simulink model "z2"  (R2023a)
settings: Solver=VariableStepAuto  StartTime=0.0  StopTime=10.0  RelTol=1e-3
libraries: fl_lib x10, nesl_utility x7, simulink_extras x2, ee_lib x2
settings Model: Creator=Artyom  LastModifiedBy=Пажылой ай3

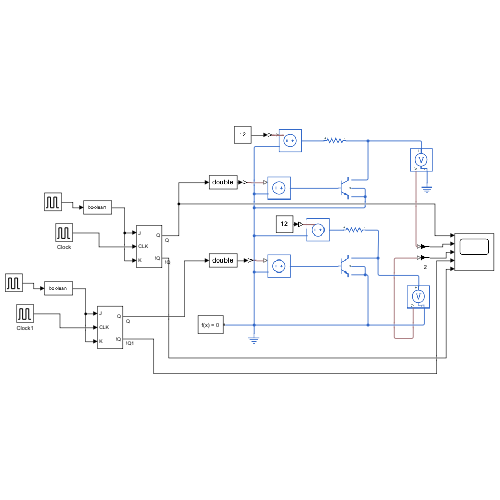
[thumbnail: Simulink's stored preview of the top-level diagram]
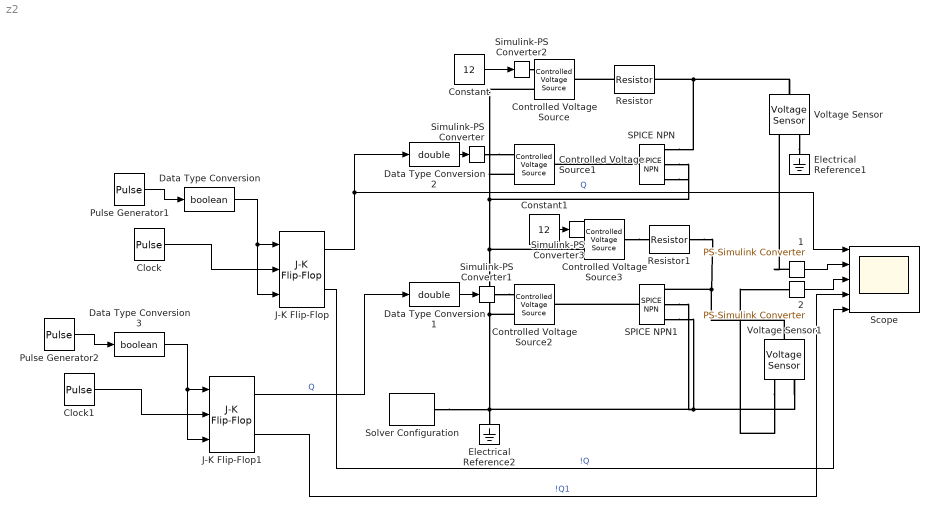
== system z2 ==
  1 : nesl_utility/PS-Simulink Converter  PhysicalDomain=network_engine_domain  SubClassName=ps_output  LeftPortType=input  RightPortType=output  PseudoPeriodic=off  Frequencies=[]  VectorFormat=inherit  Unit=inherit  AffineConversion=off
  2 : nesl_utility/PS-Simulink Converter  PhysicalDomain=network_engine_domain  SubClassName=ps_output  LeftPortType=input  RightPortType=output  PseudoPeriodic=off  Frequencies=[]  VectorFormat=inherit  Unit=inherit  AffineConversion=off
  Clock : DiscretePulseGenerator  PulseType=Time based  Period=1  PulseWidth=50
  Clock1 : DiscretePulseGenerator  PulseType=Time based  Period=1  PulseWidth=50  PhaseDelay=1
  Constant : Constant  Value=12
  Constant1 : Constant  Value=12
  Controlled Voltage Source{,1..3} (4 alike) : fl_lib/Electrical/Electrical Sources/Controlled Voltage Source
  Data Type Conversion : DataTypeConversion  OutDataTypeStr=boolean  SaturateOnIntegerOverflow=off  RndMeth=Floor
  Data Type Conversion1 : DataTypeConversion  OutDataTypeStr=double  SaturateOnIntegerOverflow=off  RndMeth=Floor
  Data Type Conversion2 : DataTypeConversion  OutDataTypeStr=double  SaturateOnIntegerOverflow=off  RndMeth=Floor
  Data Type Conversion3 : DataTypeConversion  OutDataTypeStr=boolean  SaturateOnIntegerOverflow=off  RndMeth=Floor
  Electrical Reference1 : fl_lib/Electrical/Electrical Elements/Electrical Reference
  Electrical Reference2 : fl_lib/Electrical/Electrical Elements/Electrical Reference
  J-K Flip-Flop : simulink_extras/Flip Flops/J-K Flip-Flop  initial_condition=0
  J-K Flip-Flop1 : simulink_extras/Flip Flops/J-K Flip-Flop  initial_condition=0
  Pulse Generator1 : DiscretePulseGenerator  PulseType=Time based  Period=0.035  PulseWidth=50
  Pulse Generator2 : DiscretePulseGenerator  PulseType=Time based  Period=0.035  PulseWidth=50
  Resistor : fl_lib/Electrical/Electrical Elements/Resistor  R=60 Ohm  i_specify=off  i_priority=None  i=0 A  i_nominal_specify=off  i_nominal_unit=A  i_nominal_value=1  v_specify=off  v_priority=None  v=0 V  v_nominal_specify=off  v_nominal_unit=V  v_nominal_value=1
  Resistor1 : fl_lib/Electrical/Electrical Elements/Resistor  R=60 Ohm  i_specify=off  i_priority=None  i=0 A  i_nominal_specify=off  i_nominal_unit=A  i_nominal_value=1  v_specify=off  v_priority=None  v=0 V  v_nominal_specify=off  v_nominal_unit=V  v_nominal_value=1
  SPICE NPN : ee_lib/Additional Components/SPICE Semiconductors/SPICE NPN  AREA=1.0 m^2  SCALE=1  IS=1.0e-16 A/m^2  BF=100.0  NF=1  VAF=Inf V  IKF=Inf A/m^2  ISE=0 A/m^2  NE=1.5  BR=1  NR=1  VAR=Inf V  IKR=Inf A/m^2  ISC=0 A/m^2  NC=2  RB=1 Ohm*m^2  IRB=Inf A/m^2  RBM=0 Ohm*m^2  RE=1e-4 Ohm*m^2  RC=0.01 Ohm*m^2  C_param=1  FC=0.5  IC_given=1  ICVBE=0 V  ICVCE=0 V  CJE=0 F/m^2  VJE=0.75 V  MJE=0.33  TF=0 s  XTF=0  VTF=Inf V  ITF=0 A/m^2  CJC=0 F/m^2  VJC=0.75 V  MJC=0.33  XCJC=1  TR=0 s  CJS=0 F/m^2  VJS=0.75 V  MJS=0  T_param=1  XTB=0  EG=1.11 eV  XTI=3  TFIXED=300.15 K  TMEAS=300.15 K  TOFFSET=0 K
      settings: InternalSimscapePortConfiguration="{\"Bottom\":[],\"Left\":[{\"id\":\"bx\",\"label\":\"\",\"type\":\"foundation.electrical.electrical\"}],\"Right\":[{\"id\":\"cx\",\"label\":\"\",\"type\":\"foundation.electrical.electrical\"},{\"id\":\"sx\",\"label\":\"s\",\"type\":\"foundation.electrical.electrical\"},{\"id\":\"ex\",\"label\":\"\",\"type\":\"foundation.electrical.electrical\"}],\"Top\":[]}"
  SPICE NPN1 : ee_lib/Additional Components/SPICE Semiconductors/SPICE NPN  AREA=1.0 m^2  SCALE=1  IS=1.0e-16 A/m^2  BF=100.0  NF=1  VAF=Inf V  IKF=Inf A/m^2  ISE=0 A/m^2  NE=1.5  BR=1  NR=1  VAR=Inf V  IKR=Inf A/m^2  ISC=0 A/m^2  NC=2  RB=1 Ohm*m^2  IRB=Inf A/m^2  RBM=0 Ohm*m^2  RE=1e-4 Ohm*m^2  RC=0.01 Ohm*m^2  C_param=1  FC=0.5  IC_given=1  ICVBE=0 V  ICVCE=0 V  CJE=0 F/m^2  VJE=0.75 V  MJE=0.33  TF=0 s  XTF=0  VTF=Inf V  ITF=0 A/m^2  CJC=0 F/m^2  VJC=0.75 V  MJC=0.33  XCJC=1  TR=0 s  CJS=0 F/m^2  VJS=0.75 V  MJS=0  T_param=1  XTB=0  EG=1.11 eV  XTI=3  TFIXED=300.15 K  TMEAS=300.15 K  TOFFSET=0 K
      settings: InternalSimscapePortConfiguration="{\"Bottom\":[],\"Left\":[{\"id\":\"bx\",\"label\":\"\",\"type\":\"foundation.electrical.electrical\"}],\"Right\":[{\"id\":\"cx\",\"label\":\"\",\"type\":\"foundation.electrical.electrical\"},{\"id\":\"sx\",\"label\":\"s\",\"type\":\"foundation.electrical.electrical\"},{\"id\":\"ex\",\"label\":\"\",\"type\":\"foundation.electrical.electrical\"}],\"Top\":[]}"
  Scope : Scope  NumInputPorts=5
  Simulink-PS Converter{,1..3} (4 alike) : nesl_utility/Simulink-PS Converter  PhysicalDomain=network_engine_domain  SubClassName=ps_input  LeftPortType=input  RightPortType=output  PseudoPeriodic=off  Frequencies=[]  NoiseDistribution=none  NoiseParameters=[]  Unit=1  AffineConversion=off  FilteringAndDerivatives=provide  SimscapeFilterOrder=1  InputFilterTimeConstant=0.001  UdotUserProvided=0
  Solver Configuration : nesl_utility/Solver Configuration  PhysicalDomain=network_engine_domain  SubClassName=solver  LeftPortType=input  RightPortType=generic  Tones=[]  Harmonics=[]  SimulateNoise=off  Profile=off  UseLocalSampling=off  EnableSwitchedLinearOptims=on  FrequencyDomain=off  UseCCode=off  RelTol=0.001  AbsTol=0.001  MinStep=1e-09  ToWorkspace=off  RevertToSquareIcSolve=off  NumHomotopyIterations=100  PhasorMode=off  PhasorModeNumHarmonics=1  ConsistencySolver=NEWTON_XTOL_AFTER_FTOL  IndexReductionMethod=DerivativeReplacement  DoDC=off  ResidualTolerance=1e-09  ConsistencyTolSource=GLOBAL  ConsistencyAbsTol=0.001  ConsistencyRelTol=0.001  ConsistencyTolFactor=0.001  UseLocalSolver=off  LocalSolverChoice=NE_BACKWARD_EULER_ADVANCER  ResolveIndetEquations=on  FunctionEvalNumThread=1  LocalSolverSampleTime=0.001  DoFixedCost=off  MaxNonlinIter=3  MaxModeIter=2  ComputeImpulses=off  ImpulseIterations=2  LinearAlgebra=auto  LinearAlgebraNumThread=0  EquationFormulation=NE_TIME_EF  DelaysMemoryBudget=1024  AutomaticFiltering=on  FilteringTimeConstant=0.001  PartitionStorageMethod=AS_NEEDED  PartitionMemoryBudget=1024  PartitionMethod=ROBUST
  Voltage Sensor : fl_lib/Electrical/Electrical Sensors/Voltage Sensor
  Voltage Sensor1 : fl_lib/Electrical/Electrical Sensors/Voltage Sensor
  wires:
  Clock/1 -> J-K Flip-Flop/2
  Pulse Generator1/1 -> Data Type Conversion/1
  Data Type Conversion2/1 -> Simulink-PS Converter/1
  Data Type Conversion/1 -> J-K Flip-Flop/3, J-K Flip-Flop/1
  J-K Flip-Flop/1 -> Data Type Conversion2/1, Scope/1  "Q"
  1/1 -> Scope/2
  Data Type Conversion1/1 -> Simulink-PS Converter1/1
  J-K Flip-Flop/2 -> Scope/5  "!Q"
  2/1 -> Scope/3
  Constant/1 -> Simulink-PS Converter2/1
  Constant1/1 -> Simulink-PS Converter3/1
  Data Type Conversion3/1 -> J-K Flip-Flop1/3, J-K Flip-Flop1/1
  Clock1/1 -> J-K Flip-Flop1/2
  Pulse Generator2/1 -> Data Type Conversion3/1
  J-K Flip-Flop1/1 -> Data Type Conversion1/1  "Q"
  J-K Flip-Flop1/2 -> Scope/4  "!Q1"
  connections:
  Voltage Sensor/RConn2 -- Electrical Reference1/LConn1
  Simulink-PS Converter/RConn1 -- Controlled Voltage Source1/RConn1
  SPICE NPN/LConn1 -- Controlled Voltage Source1/LConn1
  1/LConn1 -- Voltage Sensor/RConn1
  SPICE NPN1/LConn1 -- Controlled Voltage Source2/LConn1
  Simulink-PS Converter1/RConn1 -- Controlled Voltage Source2/RConn1
  Solver Configuration/RConn1 -- SPICE NPN/RConn2 -- SPICE NPN/RConn3 -- Controlled Voltage Source/RConn2 -- Controlled Voltage Source1/RConn2 -- Controlled Voltage Source3/RConn2 -- Controlled Voltage Source2/RConn2 -- Electrical Reference2/LConn1 -- SPICE NPN1/RConn2 -- SPICE NPN1/RConn3 -- Voltage Sensor1/RConn2
  Voltage Sensor1/RConn1 -- 2/LConn1
  Simulink-PS Converter3/RConn1 -- Controlled Voltage Source3/RConn1
  Simulink-PS Converter2/RConn1 -- Controlled Voltage Source/RConn1
  Resistor/LConn1 -- Controlled Voltage Source/LConn1
  Voltage Sensor1/LConn1 -- Resistor1/RConn1 -- SPICE NPN1/RConn1
  SPICE NPN/RConn1 -- Voltage Sensor/LConn1 -- Resistor/RConn1
  Controlled Voltage Source3/LConn1 -- Resistor1/LConn1
